simulink model "satellite"  (R2021b)
settings: Solver=VariableStepAuto  StartTime=0.0  StopTime=10.0  RelTol=1e-3
settings Model: Creator=DELL  LastModifiedBy=DELL

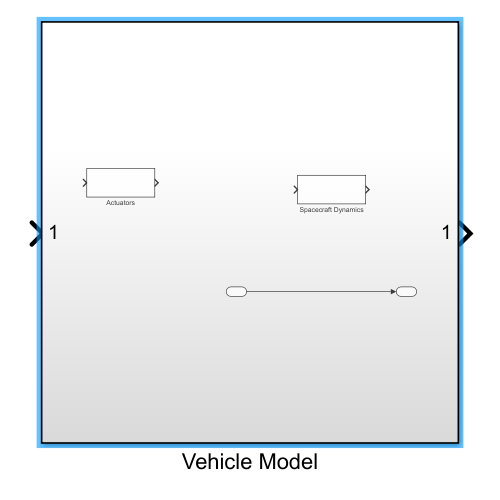
[thumbnail: Simulink's stored preview of the top-level diagram]
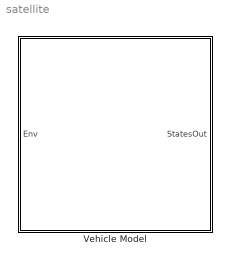
== system satellite ==
  Vehicle Model : Subsystem

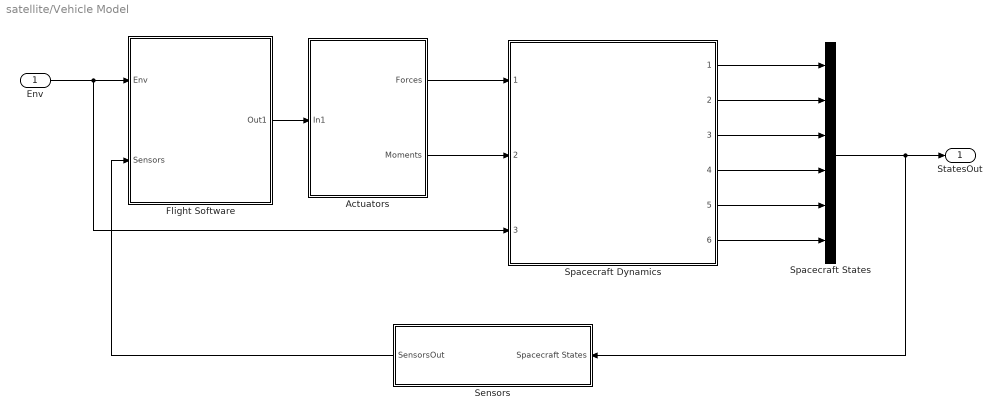
== system satellite/Vehicle Model ==
  Env : Inport
  Actuators : Subsystem
  Flight Software : Subsystem
  Sensors : Subsystem
  Spacecraft Dynamics : Subsystem  ReferencedSubsystem=Spacecraft_Dynamics  Mass=1  J=eye(3)
  Spacecraft States : Mux  Inputs=6
  StatesOut : Outport
  wires:
  Flight Software/1(Out1) -> Actuators/1(In1)
  Actuators/1(Forces) -> Spacecraft Dynamics/1
  Actuators/2(Moments) -> Spacecraft Dynamics/2
  Env/1 -> Spacecraft Dynamics/3, Flight Software/1(Env)
  Spacecraft Dynamics/1 -> Spacecraft States/1
  Spacecraft Dynamics/2 -> Spacecraft States/2
  Spacecraft Dynamics/3 -> Spacecraft States/3
  Spacecraft Dynamics/4 -> Spacecraft States/4
  Spacecraft Dynamics/5 -> Spacecraft States/5
  Spacecraft Dynamics/6 -> Spacecraft States/6
  Spacecraft States/1 -> Sensors/1(Spacecraft States), StatesOut/1
  Sensors/1(SensorsOut) -> Flight Software/2(Sensors)

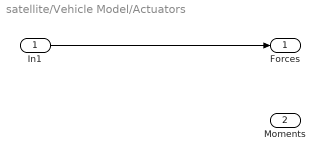
== system satellite/Vehicle Model/Actuators ==
  In1 : Inport
  Forces : Outport
  Moments : Outport  Port=2
  wires:
  In1/1 -> Forces/1

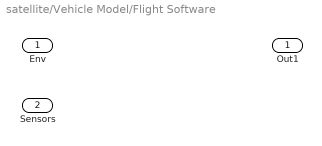
== system satellite/Vehicle Model/Flight Software ==
  Env : Inport
  Sensors : Inport  Port=2
  Out1 : Outport

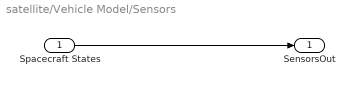
== system satellite/Vehicle Model/Sensors ==
  Spacecraft States : Inport
  SensorsOut : Outport
  wires:
  Spacecraft States/1 -> SensorsOut/1
